simulink model "motor_simulator"  (R2020b)
settings: Solver=VariableStepAuto  StartTime=0.0  StopTime=2.0  FixedStep=1e-8  RelTol=1e-3
libraries: cstblocks x2, simulink x1
settings Model: Creator=gromualdi  LastModifiedBy=gromualdi

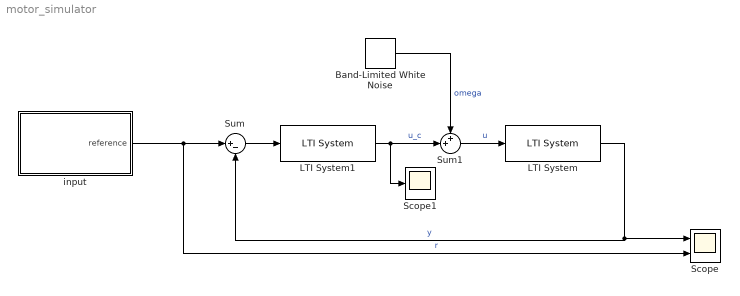
== system motor_simulator ==
  Band-Limited White Noise : simulink/Sources/Band-Limited White Noise  Cov=[0.0000001]  Ts=1e-4  seed=[23341]
  LTI System : cstblocks/LTI System  sys=G_nom  IC=[]
  LTI System1 : cstblocks/LTI System  sys=discrete_controller  IC=[]
  Scope : Scope  NumInputPorts=2
  Scope1 : Scope
  Sum : Sum  Inputs=|+-
  Sum1 : Sum  Inputs=++|
  input : Subsystem
  wires:
  LTI System/1 -> Sum/2, Scope/1  "y"
  Sum/1 -> LTI System1/1
  LTI System1/1 -> Scope1/1, Sum1/2  "u_c"
  Sum1/1 -> LTI System/1  "u"
  Band-Limited White Noise/1 -> Sum1/1  "omega"
  input/1(reference) -> Scope/2, Sum/1  "r"

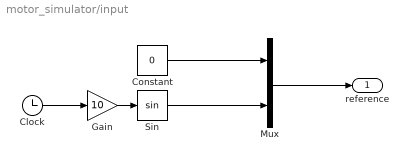
== system motor_simulator/input ==
  Clock : Clock
  Constant : Constant  Value=0
  Gain : Gain  Gain=10
  Mux : Mux  Inputs=2
  Sin : Trigonometry
  reference : Outport
  wires:
  Gain/1 -> Sin/1
  Clock/1 -> Gain/1
  Sin/1 -> Mux/2
  Constant/1 -> Mux/1
  Mux/1 -> reference/1
